simulink library "CRYP_MN_MASTER"  (Simulink 8.6)
settings: Solver=ode45  StartTime=0.0  StopTime=10.0  RelTol=1e-3
libraries: VIS_LIB x19, cdsEpicsOut x16, cdsFilt x12, cdsTP x12, cdsMuxMatrix x6, cdsEpicsBinIn x5, KAGRA_UTIL x1, cdsFunctionCall x1
(part 1 of 2)
settings Model: Creator=controls  LastModifiedBy=controls

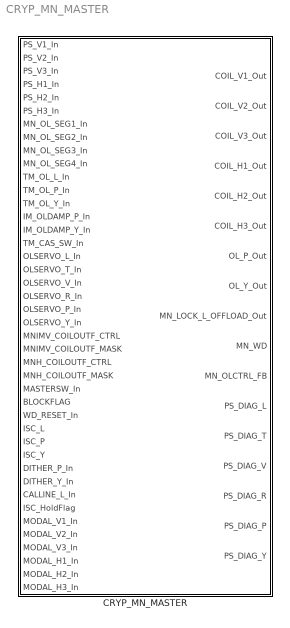
== system CRYP_MN_MASTER ==
  CRYP_MN_MASTER : Subsystem  Description=SIXOSEMSTAGE_FACE_MASTER

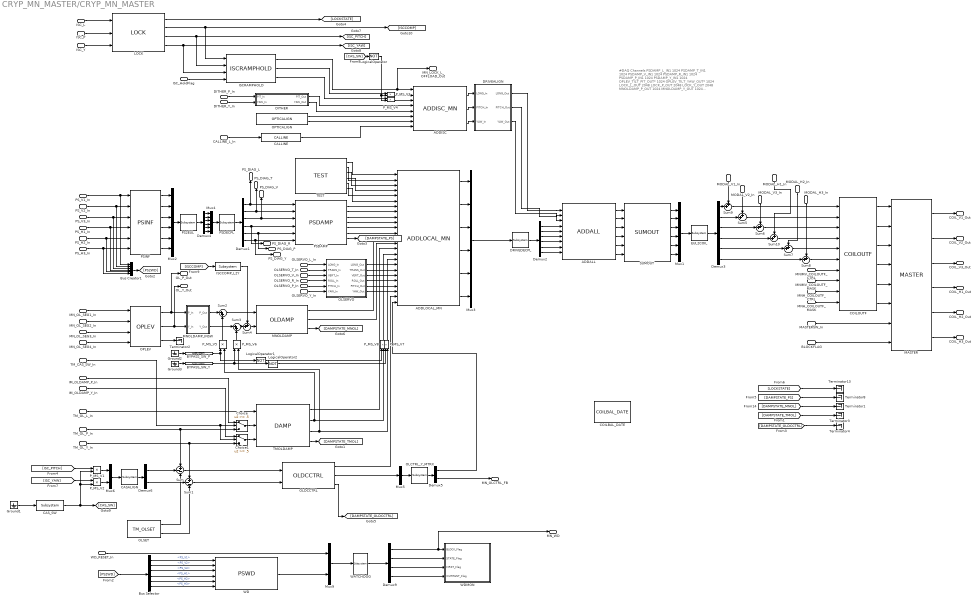
== system CRYP_MN_MASTER/CRYP_MN_MASTER ==
  note: #DAQ Channels
      | PSDAMP_L_IN1 1024
      | PSDAMP_T_IN1 1024
      | PSDAMP_V_IN1 1024
      | PSDAMP_R_IN1 1024
      | PSDAMP_P_IN1 1024
      | PSDAMP_Y_IN1 1024
      | OPLEV_TILT_PIT_OUT* 1024
      | OPLEV_TILT_YAW_OUT* 1024
      | LOCK_L_OUT 2048
      | LOCK_P_OUT 2048
      | LOCK_Y_OUT 2048
      | MNOLDAMP_P_OUT 1024
      | MNOLDAMP_Y_OUT 1024
      | TMOLDAMP_L_OUT 1024
      | TMOLDAMP_P_OUT 1024
      | TMOLDAMP_Y_OUT 1024
      | OLDCCTRL_P_OUT 256
      | OLDCCTRL_Y_OUT 256
      | PSDAMP_L_OUT 1024
      | PSDAMP_T_OUT 1024
      | PSDAMP_V_OUT 1024
      | PSDAMP_R_OUT 1024
      | PSDAMP_P_OUT 1024
      | PSDAMP_Y_OUT 1024
      | SUMOUT_L_OUT 512
      | SUMOUT_T_OUT 512
      | SUMOUT_V_OUT 512
      | SUMOUT_R_OUT 512
      | SUMOUT_P_OUT 512
      | SUMOUT_Y_OUT 512
      | MASTER_OUT_H1 1024
      | MASTER_OUT_H2 1024
      | MASTER_OUT_H3 1024
      | MASTER_OUT_V1 1024
      | MASTER_OUT_V2 1024
      | MASTER_OUT_V3 1024
  PS_V1_In : Inport
  PS_V2_In : Inport  Port=2
  PS_V3_In : Inport  Port=3
  PS_H1_In : Inport  Port=4
  PS_H2_In : Inport  Port=5
  PS_H3_In : Inport  Port=6
  MN_OL_SEG1_In : Inport  Port=7
  MN_OL_SEG2_In : Inport  Port=8
  MN_OL_SEG3_In : Inport  Port=9
  MN_OL_SEG4_In : Inport  Port=10
  TM_OL_L_In : Inport  Port=11
  TM_OL_P_In : Inport  Port=12
  TM_OL_Y_In : Inport  Port=13
  IM_OLDAMP_P_In : Inport  Port=14
  IM_OLDAMP_Y_In : Inport  Port=15
  TM_CAS_SW_In : Inport  Port=16
  OLSERVO_L_In : Inport  Port=17
  OLSERVO_T_In : Inport  Port=18
  OLSERVO_V_In : Inport  Port=19
  OLSERVO_R_In : Inport  Port=20
  OLSERVO_P_In : Inport  Port=21
  OLSERVO_Y_In : Inport  Port=22
  MNIMV_COILOUTF_CTRL : Inport  Port=23
  MNIMV_COILOUTF_MASK : Inport  Port=24
  MNH_COILOUTF_CTRL : Inport  Port=25
  MNH_COILOUTF_MASK : Inport  Port=26
  MASTERSW_In : Inport  Port=27
  BLOCKFLAG : Inport  Port=28
  WD_RESET_In : Inport  Port=29
  ISC_L : Inport  Port=30
  ISC_P : Inport  Port=31
  ISC_Y : Inport  Port=32
  DITHER_P_In : Inport  Port=33
  DITHER_Y_In : Inport  Port=34
  CALLINE_L_In : Inport  Port=35
  ISC_HoldFlag : Inport  Port=36
  MODAL_V1_In : Inport  Port=37
  MODAL_V2_In : Inport  Port=38
  MODAL_V3_In : Inport  Port=39
  MODAL_H1_In : Inport  Port=40
  MODAL_H2_In : Inport  Port=41
  MODAL_H3_In : Inport  Port=42
  ADDALL : VIS_LIB/CrypParts/ADDALL
  ADDISC : VIS_LIB/CrypParts/ADDISC_MN
  ADDLOCAL_MN : VIS_LIB/CrypParts/ADDLOCAL_MN
  BYPASS_SW_P : cdsEpicsBinIn/Subsystem  Tag=cdsEpicsBinIn  Description=|
      | Purpose:                                                                            
      | Create an EPICS binary (0 or 1) input channel to the FE realtime controls.          
      |                                                                                     
      | Operation:                                                                          
      | Outputs value from an EPICS ai record. Value is binary input (bi Epics record type).
      |                                                                                     
      | Usage:                                                                              
      | Name the part with the desired EPICS channel name.
      settings: AttributesFormatString=%<Tag>
  BYPASS_SW_Y : cdsEpicsBinIn/Subsystem  Tag=cdsEpicsBinIn  Description=|
      | Purpose:                                                                            
      | Create an EPICS binary (0 or 1) input channel to the FE realtime controls.          
      |                                                                                     
      | Operation:                                                                          
      | Outputs value from an EPICS ai record. Value is binary input (bi Epics record type).
      |                                                                                     
      | Usage:                                                                              
      | Name the part with the desired EPICS channel name.
      settings: AttributesFormatString=%<Tag>
  Bus Creator1 : BusCreator  Inputs='PS_V1','PS_V2','PS_V3','PS_H1','PS_H2','PS_H3'
  Bus Selector : BusSelector  OutputSignals=PS_V1,PS_V2,PS_V3,PS_H1,PS_H2,PS_H3
  CALLINE : VIS_LIB/CALLINE
  CASALIGN : cdsMuxMatrix/Subsystem  Tag=cdsMuxMatrix  Description=Any size matrix. Inputs and outputs must be connected using Mux and Demux parts.
      settings: AttributesFormatString=%<Tag>
  CAS_SW : cdsEpicsBinIn/Subsystem  Tag=cdsEpicsBinIn  Description=|
      | Purpose:                                                                            
      | Create an EPICS binary (0 or 1) input channel to the FE realtime controls.          
      |                                                                                     
      | Operation:                                                                          
      | Outputs value from an EPICS ai record. Value is binary input (bi Epics record type).
      |                                                                                     
      | Usage:                                                                              
      | Name the part with the desired EPICS channel name.
      settings: AttributesFormatString=%<Tag>
  COILBAL_DATE : VIS_LIB/COILBAL_DATE
  COILOUTF : VIS_LIB/CRYp Blocks/COILOUTF
  Choice : Switch  Threshold=.5
  Choice1 : Switch  Threshold=.5
  DITHER : Subsystem
  DRIVEALIGN : Subsystem
  DRIVEDECPL : cdsMuxMatrix/Subsystem  Tag=cdsMuxMatrix  Description=Any size matrix. Inputs and outputs must be connected using Mux and Demux parts.
      settings: AttributesFormatString=%<Tag>
  Demux{1..4} (4 alike) : Demux  Outputs=6
  Demux5 : Demux  Outputs=2
  Demux6 : Demux  Outputs=2
  Demux9 : Demux
  EUL2COIL : cdsMuxMatrix/Subsystem  Tag=cdsMuxMatrix  Description=Any size matrix. Inputs and outputs must be connected using Mux and Demux parts.
      settings: AttributesFormatString=%<Tag>
  Ground1 : Ground
  Ground2 : Ground
  Ground3 : Ground
  ISCCOMP_L2Y : cdsFilt/Subsystem  Tag=cdsFilt  Description=|
      | Purpose:                                                                                                                                                                                                                                  
      | Standard CDS IIR filter module.                                                                                                                                                                                                           
      |                                                                                                                                                                                                                                           
      | Operation:                                                                                                                                                                                                                                
      | Consists of 10 second order section IIR filters, plus a ramped gain stage. In FE code, also provides pre-defined test points and excitation channel inputs. The filter coefficients are defined in the LIGO system using the 'foton' tool.
      |                                                                                                                                                                                                                                           
      | Usage:                                                                                                                                                                                                                                    
      | Name the part with the desired filter module name.
      settings: AttributesFormatString=%<Tag>
  ISCRAMPHOLD : KAGRA_UTIL/ISCRAMPHOLD
  LOCK : VIS_LIB/CrypParts/LOCK
  LogicalOperator : Logic  Operator=NOT  AllPortsSameDT=off  OutDataTypeStr=boolean
  LogicalOperator1 : Logic  Operator=NOT  AllPortsSameDT=off  OutDataTypeStr=boolean
  LogicalOperator2 : Logic  Operator=NOT  AllPortsSameDT=off  OutDataTypeStr=boolean
  MASTER : VIS_LIB/CRYp Blocks/MASTER
  MNOLDAMP : VIS_LIB/OLDAMP
  MNOLDAMP_INSW : Subsystem
  Mux{1..4} (4 alike) : Mux  Inputs=6
  Mux5 : Mux  Inputs=1
  Mux6 : Mux  Inputs=2
  Mux9 : Mux  Inputs=2
  OLCTRL_Y_MTRX : cdsMuxMatrix/Subsystem  Tag=cdsMuxMatrix  Description=Any size matrix. Inputs and outputs must be connected using Mux and Demux parts.
      settings: AttributesFormatString=%<Tag>
  OLDCCTRL : VIS_LIB/CrypParts/OLDCCTRL
  OLSERVO : Subsystem
  OLSET : VIS_LIB/CrypParts/TM_OLSET
  OPLEV : VIS_LIB/CrypParts/OPLEV
  OPTICALIGN : VIS_LIB/CrypParts/OPTICALIGN
  PS2EUL : cdsMuxMatrix/Subsystem  Tag=cdsMuxMatrix  Description=Any size matrix. Inputs and outputs must be connected using Mux and Demux parts.
      settings: AttributesFormatString=%<Tag>
  PSDAMP : VIS_LIB/CrypParts/PSDAMP
  PSDECPL : cdsMuxMatrix/Subsystem  Tag=cdsMuxMatrix  Description=Any size matrix. Inputs and outputs must be connected using Mux and Demux parts.
      settings: AttributesFormatString=%<Tag>
  PSINF : VIS_LIB/CrypParts/PSINF
  P_MS_V{1..8} (8 alike) : Product  RndMeth=Zero
  SUMOUT : VIS_LIB/CrypParts/SUMOUT
  Sum : Sum  Inputs=+--
  Sum1 : Sum  Inputs=+--
  Sum{4..10} (7 alike) : Sum  Inputs=++|
  Sum2 : Sum  Inputs=|++
  Sum3 : Sum  Inputs=|++
  TEST : VIS_LIB/CrypParts/TEST
  TMOLDAMP : VIS_LIB/CrypParts/DAMP
  Terminator{1..4,8,13} (6 alike) : Terminator
  WATCHDOG : cdsFunctionCall/Subsystem  Tag=cdsFunctionCall  Description=inline OSEMWATCHDOG /opt/rtcds/userapps/release/vis/common/src/WATCHDOG.c
      settings: AttributesFormatString=%<Tag>\n%<Description>
  WD : VIS_LIB/CRYp Blocks/PSWD
  WDMON : Subsystem
  COIL_V1_Out : Outport
  COIL_V2_Out : Outport  Port=2
  COIL_V3_Out : Outport  Port=3
  COIL_H1_Out : Outport  Port=4
  COIL_H2_Out : Outport  Port=5
  COIL_H3_Out : Outport  Port=6
  OL_P_Out : Outport  Port=7
  OL_Y_Out : Outport  Port=8
  MN_LOCK_L_OFFLOAD_Out : Outport  Port=9
  MN_WD : Outport  Port=10
  MN_OLCTRL_FB : Outport  Port=11
  PS_DIAG_L : Outport  Port=12
  PS_DIAG_T : Outport  Port=13
  PS_DIAG_V : Outport  Port=14
  PS_DIAG_R : Outport  Port=15
  PS_DIAG_P : Outport  Port=16
  PS_DIAG_Y : Outport  Port=17
  wires:
  Demux3/6 -> Sum8/2
  MODAL_H3_In/1 -> Sum8/1
  Sum8/1 -> COILOUTF/6
  Demux3/5 -> Sum7/2
  MODAL_H2_In/1 -> Sum7/1
  Sum7/1 -> COILOUTF/5
  Demux3/4 -> Sum10/2
  MODAL_H1_In/1 -> Sum10/1
  Sum10/1 -> COILOUTF/4
  Demux3/3 -> Sum6/2
  MODAL_V3_In/1 -> Sum6/1
  Sum6/1 -> COILOUTF/3
  Demux3/2 -> Sum5/2
  MODAL_V2_In/1 -> Sum5/1
  Sum5/1 -> COILOUTF/2
  Demux3/1 -> Sum9/2
  MODAL_V1_In/1 -> Sum9/1
  Sum9/1 -> COILOUTF/1
  Demux1/1 -> PSDAMP/1, PS_DIAG_L/1
  Demux1/2 -> PSDAMP/2, PS_DIAG_T/1
  Demux1/5 -> PSDAMP/5, PS_DIAG_P/1
  Demux1/6 -> PSDAMP/6, PS_DIAG_Y/1
  ADDLOCAL_MN/6 -> Mux3/6
  ADDLOCAL_MN/5 -> Mux3/5
  ADDLOCAL_MN/4 -> Mux3/4
  ADDLOCAL_MN/3 -> Mux3/3
  ADDLOCAL_MN/2 -> Mux3/2
  ADDLOCAL_MN/1 -> Mux3/1
  ISC_HoldFlag/1 -> ISCRAMPHOLD/4
  ISCRAMPHOLD/3 -> P_MS_V4/1
  ISCRAMPHOLD/2 -> P_MS_V3/1
  ISCRAMPHOLD/1 -> ADDISC/1, MN_LOCK_L_OFFLOAD_Out/1
  MNOLDAMP_INSW/2(Y_Out) -> Sum3/1
  MNOLDAMP_INSW/1(P_Out) -> Sum2/1
  P_MS_V7/1 -> ADDLOCAL_MN/17
  P_MS_V8/1 -> ADDLOCAL_MN/16
  LogicalOperator1/1 -> P_MS_V8/1
  TM_CAS_SW_In/1 -> Choice/2, Choice1/2
  IM_OLDAMP_Y_In/1 -> Choice1/1
  IM_OLDAMP_P_In/1 -> Choice/1
  P_MS_V6/1 -> Sum3/2
  P_MS_V5/1 -> Sum2/2
  Sum2/1 -> MNOLDAMP/1
  Choice1/1 -> TMOLDAMP/3
  Choice/1 -> TMOLDAMP/2
  OLSET/2 -> Sum1/3
  OLSET/1 -> Sum/3
  Demux6/2 -> Sum1/2
  Demux6/1 -> Sum/2
  LogicalOperator/1 -> P_MS_V4/2, P_MS_V3/2
  P_MS_V3/1 -> ADDISC/2
  P_MS_V4/1 -> ADDISC/3
  DRIVEALIGN/3(YAW_Out) -> ADDALL/3
  DRIVEALIGN/2(PITCH_Out) -> ADDALL/2
  [CAS_SW] -> LogicalOperator/1
  CASALIGN/1 -> Demux6/1
  Mux6/1 -> CASALIGN/1
  P_MS_V2/1 -> Mux6/2
  P_MS_V1/1 -> Mux6/1
  CAS_SW/1 -> P_MS_V2/2, P_MS_V1/2, [CAS_SW]
  [ISC_PITCH] -> P_MS_V1/1
  [ISC_YAW] -> P_MS_V2/1
  Ground1/1 -> CAS_SW/1
  Demux5/1 -> ADDLOCAL_MN/25
  OLDCCTRL/2 -> Mux5/1
  Demux5/2 -> MN_OLCTRL_FB/1
  OLCTRL_Y_MTRX/1 -> Demux5/1
  Mux5/1 -> OLCTRL_Y_MTRX/1
  Sum1/1 -> OLDCCTRL/2
  Sum/1 -> OLDCCTRL/1
  [DAMPSTATE_OLDCCTRL] -> Terminator4/1
  OLDCCTRL/1 -> ADDLOCAL_MN/24
  TEST/6 -> ADDLOCAL_MN/6
  TEST/5 -> ADDLOCAL_MN/5
  TEST/4 -> ADDLOCAL_MN/4
  TEST/3 -> ADDLOCAL_MN/3
  TEST/2 -> ADDLOCAL_MN/2
  TEST/1 -> ADDLOCAL_MN/1
  OLDCCTRL/3 -> [DAMPSTATE_OLDCCTRL]
  OLSERVO/3(VERT_Out) -> ADDLOCAL_MN/20
  OLSERVO/2(TRANS_Out) -> ADDLOCAL_MN/19
  OLSERVO/1(LONG_Out) -> ADDLOCAL_MN/18
  OLSERVO/6(YAW_Out) -> ADDLOCAL_MN/23
  OLSERVO/5(PITCH_Out) -> ADDLOCAL_MN/22
  OLSERVO/4(ROLL_Out) -> ADDLOCAL_MN/21
  OLSERVO_Y_In/1 -> OLSERVO/6(YAW_In)
  OLSERVO_P_In/1 -> OLSERVO/5(PITCH_In)
  OLSERVO_R_In/1 -> OLSERVO/4(ROLL_In)
  OLSERVO_V_In/1 -> OLSERVO/3(VERT_In)
  OLSERVO_T_In/1 -> OLSERVO/2(TRANS_In)
  OLSERVO_L_In/1 -> OLSERVO/1(LONG_In)
  PSDECPL/1 -> Demux1/1
  Mux4/1 -> PSDECPL/1
  Demux4/6 -> Mux4/6
  Demux4/5 -> Mux4/5
  Demux4/4 -> Mux4/4
  Demux4/3 -> Mux4/3
  Demux4/2 -> Mux4/2
  Demux4/1 -> Mux4/1
  PS2EUL/1 -> Demux4/1
  SUMOUT/6 -> Mux1/6
  SUMOUT/5 -> Mux1/5
  SUMOUT/4 -> Mux1/4
  SUMOUT/3 -> Mux1/3
  SUMOUT/2 -> Mux1/2
  SUMOUT/1 -> Mux1/1
  ADDALL/6 -> SUMOUT/6
  ADDALL/5 -> SUMOUT/5
  ADDALL/4 -> SUMOUT/4
  ADDALL/3 -> SUMOUT/3
  ADDALL/2 -> SUMOUT/2
  ADDALL/1 -> SUMOUT/1
  TM_OL_Y_In/1 -> Choice1/3, Sum1/1
  TM_OL_P_In/1 -> Sum/1, Choice/3
  TM_OL_L_In/1 -> TMOLDAMP/1
  [DAMPSTATE_TMOL] -> Terminator3/1
  TMOLDAMP/4 -> [DAMPSTATE_TMOL]
  Demux2/3 -> ADDALL/6
  Demux2/5 -> ADDALL/8
  Demux2/4 -> ADDALL/7
  Demux2/2 -> ADDALL/5
  Demux2/6 -> ADDALL/9
  Demux2/1 -> ADDALL/4
  DRIVEDECPL/1 -> Demux2/1
  Mux3/1 -> DRIVEDECPL/1
  DRIVEALIGN/1(LONG_Out) -> ADDALL/1
  TMOLDAMP/1 -> ADDLOCAL_MN/15
  TMOLDAMP/2 -> P_MS_V5/2, P_MS_V8/2
  TMOLDAMP/3 -> P_MS_V6/2, P_MS_V7/2
  MNOLDAMP/1 -> ADDLOCAL_MN/13
  MNOLDAMP/2 -> ADDLOCAL_MN/14
  PSDAMP/6 -> ADDLOCAL_MN/12
  PSDAMP/5 -> ADDLOCAL_MN/11
  PSDAMP/4 -> ADDLOCAL_MN/10
  PSDAMP/3 -> ADDLOCAL_MN/9
  PSDAMP/2 -> ADDLOCAL_MN/8
  PSDAMP/1 -> ADDLOCAL_MN/7
  ADDISC/1 -> DRIVEALIGN/1(LONG_In)
  ADDISC/2 -> DRIVEALIGN/2(PITCH_In)
  ADDISC/3 -> DRIVEALIGN/3(YAW_In)
  OPTICALIGN/2 -> ADDISC/7
  OPTICALIGN/1 -> ADDISC/6
  DITHER/2(YAW_Out) -> ADDISC/5
  DITHER/1(PIT_Out) -> ADDISC/4
  LOCK/2 -> [ISCCOMP], ISCRAMPHOLD/1
  LOCK/3 -> [ISC_PITCH], ISCRAMPHOLD/2
  LOCK/4 -> [ISC_YAW], ISCRAMPHOLD/3
  BLOCKFLAG/1 -> MASTER/8
  Mux1/1 -> EUL2COIL/1
  Bus Selector/1 -> WD/1  "<PS_V1>"
  Bus Selector/3 -> WD/3  "<PS_V3>"
  Bus Selector/4 -> WD/4  "<PS_H1>"
  Bus Selector/5 -> WD/5  "<PS_H2>"
  Bus Selector/2 -> WD/2  "<PS_V2>"
  Bus Selector/6 -> WD/6  "<PS_H3>"
  OPLEV/3 -> Terminator2/1
  OPLEV/2 -> OL_Y_Out/1, MNOLDAMP_INSW/2(Y_In)
  OPLEV/1 -> MNOLDAMP_INSW/1(P_In), OL_P_Out/1
  MN_OL_SEG1_In/1 -> OPLEV/1
  MN_OL_SEG2_In/1 -> OPLEV/2
  MN_OL_SEG3_In/1 -> OPLEV/3
  MN_OL_SEG4_In/1 -> OPLEV/4
  ISC_L/1 -> LOCK/1
  ISC_Y/1 -> LOCK/3
  ISC_P/1 -> LOCK/2
  Demux1/3 -> PSDAMP/3, PS_DIAG_V/1
  Demux1/4 -> PSDAMP/4, PS_DIAG_R/1
  PSINF/5 -> Mux2/5
  PSINF/4 -> Mux2/4
  PSINF/3 -> Mux2/3
  PSINF/2 -> Mux2/2
  PSINF/1 -> Mux2/1
  PSINF/6 -> Mux2/6
  MASTER/3 -> COIL_V3_Out/1
  MASTER/6 -> COIL_H3_Out/1
  MASTER/5 -> COIL_H2_Out/1
  MASTER/4 -> COIL_H1_Out/1
  MASTER/2 -> COIL_V2_Out/1
  MASTER/1 -> COIL_V1_Out/1
  MASTERSW_In/1 -> MASTER/7
  COILOUTF/6 -> MASTER/6
  COILOUTF/5 -> MASTER/5
  COILOUTF/4 -> MASTER/4
  COILOUTF/3 -> MASTER/3
  COILOUTF/1 -> MASTER/1
  COILOUTF/2 -> MASTER/2
  MNH_COILOUTF_CTRL/1 -> COILOUTF/9
  MNIMV_COILOUTF_MASK/1 -> COILOUTF/8
  MNH_COILOUTF_MASK/1 -> COILOUTF/10
  MNIMV_COILOUTF_CTRL/1 -> COILOUTF/7
  PS_V3_In/1 -> PSINF/3, Bus Creator1/3
  PS_H1_In/1 -> PSINF/4, Bus Creator1/4
  PS_V2_In/1 -> PSINF/2, Bus Creator1/2
  PS_V1_In/1 -> Bus Creator1/1, PSINF/1
  PS_H3_In/1 -> PSINF/6, Bus Creator1/6
  PS_H2_In/1 -> PSINF/5, Bus Creator1/5
  [DAMPSTATE_MNOL] -> Terminator1/1
  MNOLDAMP/3 -> [DAMPSTATE_MNOL]
  DITHER_P_In/1 -> DITHER/1(PIT_In)
  DITHER_Y_In/1 -> DITHER/2(YAW_In)
  WD_RESET_In/1 -> Mux9/1
  WD/1 -> Mux9/2
  [LOCKSTATE] -> Terminator13/1
  LOCK/1 -> [LOCKSTATE]
  [DAMPSTATE_PS] -> Terminator8/1
  PSDAMP/7 -> [DAMPSTATE_PS]
  Demux9/1 -> WDMON/1(BLOCK_Flag), MN_WD/1
  Mux2/1 -> PS2EUL/1
  Bus Creator1/1 -> [PS2WD]
  [PS2WD] -> Bus Selector/1
  EUL2COIL/1 -> Demux3/1
  Demux9/2 -> WDMON/2(STATE_Flag)
  Demux9/3 -> WDMON/3(FIRST_Flag)
  Demux9/4 -> WDMON/4(CURRENT_Flag)
  Mux9/1 -> WATCHDOG/1
  WATCHDOG/1 -> Demux9/1
  Ground2/1 -> BYPASS_SW_P/1
  BYPASS_SW_P/1 -> LogicalOperator1/1, P_MS_V5/1
  LogicalOperator2/1 -> P_MS_V7/1
  BYPASS_SW_Y/1 -> P_MS_V6/1, LogicalOperator2/1
  Ground3/1 -> BYPASS_SW_Y/1
  Sum3/1 -> Sum4/2
  Sum4/1 -> MNOLDAMP/2
  ISCCOMP_L2Y/1 -> Sum4/1
  [ISCCOMP] -> ISCCOMP_L2Y/1
  CALLINE/1 -> ADDISC/8
  CALLINE_L_In/1 -> CALLINE/1

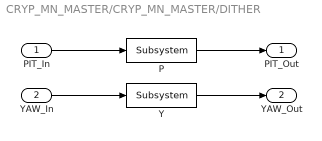
== system CRYP_MN_MASTER/CRYP_MN_MASTER/DITHER ==
  PIT_In : Inport
  YAW_In : Inport  Port=2
  P : cdsFilt/Subsystem  Tag=cdsFilt  Description=|
      | Purpose:                                                                                                                                                                                                                                  
      | Standard CDS IIR filter module.                                                                                                                                                                                                           
      |                                                                                                                                                                                                                                           
      | Operation:                                                                                                                                                                                                                                
      | Consists of 10 second order section IIR filters, plus a ramped gain stage. In FE code, also provides pre-defined test points and excitation channel inputs. The filter coefficients are defined in the LIGO system using the 'foton' tool.
      |                                                                                                                                                                                                                                           
      | Usage:                                                                                                                                                                                                                                    
      | Name the part with the desired filter module name.
      settings: AttributesFormatString=%<Tag>
  Y : cdsFilt/Subsystem  Tag=cdsFilt  Description=|
      | Purpose:                                                                                                                                                                                                                                  
      | Standard CDS IIR filter module.                                                                                                                                                                                                           
      |                                                                                                                                                                                                                                           
      | Operation:                                                                                                                                                                                                                                
      | Consists of 10 second order section IIR filters, plus a ramped gain stage. In FE code, also provides pre-defined test points and excitation channel inputs. The filter coefficients are defined in the LIGO system using the 'foton' tool.
      |                                                                                                                                                                                                                                           
      | Usage:                                                                                                                                                                                                                                    
      | Name the part with the desired filter module name.
      settings: AttributesFormatString=%<Tag>
  PIT_Out : Outport
  YAW_Out : Outport  Port=2
  wires:
  P/1 -> PIT_Out/1
  YAW_In/1 -> Y/1
  Y/1 -> YAW_Out/1
  PIT_In/1 -> P/1

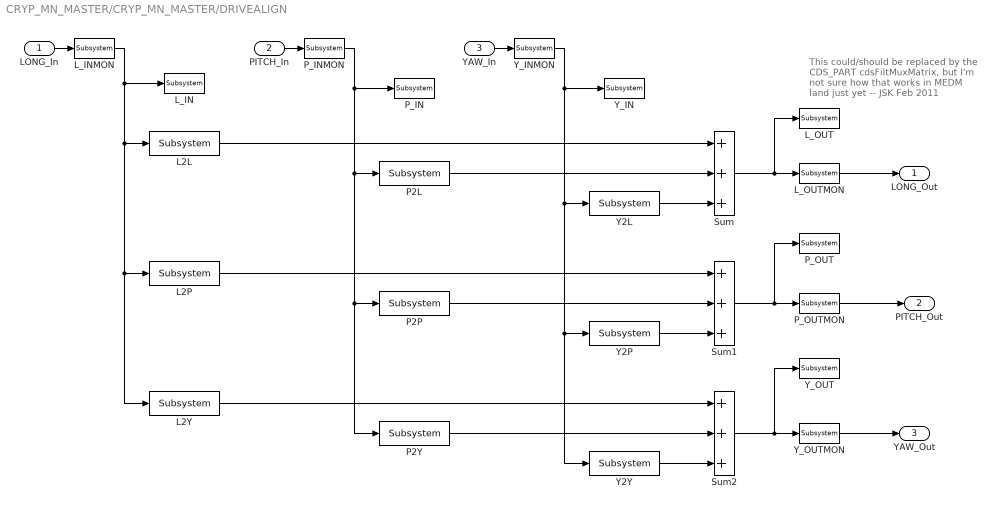
== system CRYP_MN_MASTER/CRYP_MN_MASTER/DRIVEALIGN ==
  note: This could/should be replaced by
      | the CDS_PART cdsFiltMuxMatrix,
      | but I'm not sure how that works
      | in MEDM land just yet
      | -- JSK Feb 2011
  LONG_In : Inport
  PITCH_In : Inport  Port=2
  YAW_In : Inport  Port=3
  L2L : cdsFilt/Subsystem  Tag=cdsFilt  Description=|
      | Purpose:                                                                                                                                                                                                                                  
      | Standard CDS IIR filter module.                                                                                                                                                                                                           
      |                                                                                                                                                                                                                                           
      | Operation:                                                                                                                                                                                                                                
      | Consists of 10 second order section IIR filters, plus a ramped gain stage. In FE code, also provides pre-defined test points and excitation channel inputs. The filter coefficients are defined in the LIGO system using the 'foton' tool.
      |                                                                                                                                                                                                                                           
      | Usage:                                                                                                                                                                                                                                    
      | Name the part with the desired filter module name.
      settings: AttributesFormatString=%<Tag>
  L2P : cdsFilt/Subsystem  Tag=cdsFilt  Description=|
      | Purpose:                                                                                                                                                                                                                                  
      | Standard CDS IIR filter module.                                                                                                                                                                                                           
      |                                                                                                                                                                                                                                           
      | Operation:                                                                                                                                                                                                                                
      | Consists of 10 second order section IIR filters, plus a ramped gain stage. In FE code, also provides pre-defined test points and excitation channel inputs. The filter coefficients are defined in the LIGO system using the 'foton' tool.
      |                                                                                                                                                                                                                                           
      | Usage:                                                                                                                                                                                                                                    
      | Name the part with the desired filter module name.
      settings: AttributesFormatString=%<Tag>
  L2Y : cdsFilt/Subsystem  Tag=cdsFilt  Description=|
      | Purpose:                                                                                                                                                                                                                                  
      | Standard CDS IIR filter module.                                                                                                                                                                                                           
      |                                                                                                                                                                                                                                           
      | Operation:                                                                                                                                                                                                                                
      | Consists of 10 second order section IIR filters, plus a ramped gain stage. In FE code, also provides pre-defined test points and excitation channel inputs. The filter coefficients are defined in the LIGO system using the 'foton' tool.
      |                                                                                                                                                                                                                                           
      | Usage:                                                                                                                                                                                                                                    
      | Name the part with the desired filter module name.
      settings: AttributesFormatString=%<Tag>
  L_IN : cdsTP/Subsystem  Tag=Test Point
      settings: AttributesFormatString=%<Tag>
  L_INMON : cdsEpicsOut/Subsystem  Tag=cdsEpicsOutput  Description=|
      | Purpose:                                          
      | Output a FE signal to an EPICS channel.           
      |                                                   
      | Operation:                                        
      | Takes input value and passes it to EPICS record.  
      |                                                   
      | Usage:                                            
      | Name the part with the desired EPICS rrecord name.
      settings: AttributesFormatString=%<Tag>
  L_OUT : cdsTP/Subsystem  Tag=Test Point
      settings: AttributesFormatString=%<Tag>
  L_OUTMON : cdsEpicsOut/Subsystem  Tag=cdsEpicsOutput  Description=|
      | Purpose:                                          
      | Output a FE signal to an EPICS channel.           
      |                                                   
      | Operation:                                        
      | Takes input value and passes it to EPICS record.  
      |                                                   
      | Usage:                                            
      | Name the part with the desired EPICS rrecord name.
      settings: AttributesFormatString=%<Tag>
  P2L : cdsFilt/Subsystem  Tag=cdsFilt  Description=|
      | Purpose:                                                                                                                                                                                                                                  
      | Standard CDS IIR filter module.                                                                                                                                                                                                           
      |                                                                                                                                                                                                                                           
      | Operation:                                                                                                                                                                                                                                
      | Consists of 10 second order section IIR filters, plus a ramped gain stage. In FE code, also provides pre-defined test points and excitation channel inputs. The filter coefficients are defined in the LIGO system using the 'foton' tool.
      |                                                                                                                                                                                                                                           
      | Usage:                                                                                                                                                                                                                                    
      | Name the part with the desired filter module name.
      settings: AttributesFormatString=%<Tag>
  P2P : cdsFilt/Subsystem  Tag=cdsFilt  Description=|
      | Purpose:                                                                                                                                                                                                                                  
      | Standard CDS IIR filter module.                                                                                                                                                                                                           
      |                                                                                                                                                                                                                                           
      | Operation:                                                                                                                                                                                                                                
      | Consists of 10 second order section IIR filters, plus a ramped gain stage. In FE code, also provides pre-defined test points and excitation channel inputs. The filter coefficients are defined in the LIGO system using the 'foton' tool.
      |                                                                                                                                                                                                                                           
      | Usage:                                                                                                                                                                                                                                    
      | Name the part with the desired filter module name.
      settings: AttributesFormatString=%<Tag>
  P2Y : cdsFilt/Subsystem  Tag=cdsFilt  Description=|
      | Purpose:                                                                                                                                                                                                                                  
      | Standard CDS IIR filter module.                                                                                                                                                                                                           
      |                                                                                                                                                                                                                                           
      | Operation:                                                                                                                                                                                                                                
      | Consists of 10 second order section IIR filters, plus a ramped gain stage. In FE code, also provides pre-defined test points and excitation channel inputs. The filter coefficients are defined in the LIGO system using the 'foton' tool.
      |                                                                                                                                                                                                                                           
      | Usage:                                                                                                                                                                                                                                    
      | Name the part with the desired filter module name.
      settings: AttributesFormatString=%<Tag>
  P_IN : cdsTP/Subsystem  Tag=Test Point
      settings: AttributesFormatString=%<Tag>
  P_INMON : cdsEpicsOut/Subsystem  Tag=cdsEpicsOutput  Description=|
      | Purpose:                                          
      | Output a FE signal to an EPICS channel.           
      |                                                   
      | Operation:                                        
      | Takes input value and passes it to EPICS record.  
      |                                                   
      | Usage:                                            
      | Name the part with the desired EPICS rrecord name.
      settings: AttributesFormatString=%<Tag>
  P_OUT : cdsTP/Subsystem  Tag=Test Point
      settings: AttributesFormatString=%<Tag>
  P_OUTMON : cdsEpicsOut/Subsystem  Tag=cdsEpicsOutput  Description=|
      | Purpose:                                          
      | Output a FE signal to an EPICS channel.           
      |                                                   
      | Operation:                                        
      | Takes input value and passes it to EPICS record.  
      |                                                   
      | Usage:                                            
      | Name the part with the desired EPICS rrecord name.
      settings: AttributesFormatString=%<Tag>
  Sum : Sum  Inputs=+++
  Sum1 : Sum  Inputs=+++
  Sum2 : Sum  Inputs=+++
  Y2L : cdsFilt/Subsystem  Tag=cdsFilt  Description=|
      | Purpose:                                                                                                                                                                                                                                  
      | Standard CDS IIR filter module.                                                                                                                                                                                                           
      |                                                                                                                                                                                                                                           
      | Operation:                                                                                                                                                                                                                                
      | Consists of 10 second order section IIR filters, plus a ramped gain stage. In FE code, also provides pre-defined test points and excitation channel inputs. The filter coefficients are defined in the LIGO system using the 'foton' tool.
      |                                                                                                                                                                                                                                           
      | Usage:                                                                                                                                                                                                                                    
      | Name the part with the desired filter module name.
      settings: AttributesFormatString=%<Tag>
  Y2P : cdsFilt/Subsystem  Tag=cdsFilt  Description=|
      | Purpose:                                                                                                                                                                                                                                  
      | Standard CDS IIR filter module.                                                                                                                                                                                                           
      |                                                                                                                                                                                                                                           
      | Operation:                                                                                                                                                                                                                                
      | Consists of 10 second order section IIR filters, plus a ramped gain stage. In FE code, also provides pre-defined test points and excitation channel inputs. The filter coefficients are defined in the LIGO system using the 'foton' tool.
      |                                                                                                                                                                                                                                           
      | Usage:                                                                                                                                                                                                                                    
      | Name the part with the desired filter module name.
      settings: AttributesFormatString=%<Tag>
  Y2Y : cdsFilt/Subsystem  Tag=cdsFilt  Description=|
      | Purpose:                                                                                                                                                                                                                                  
      | Standard CDS IIR filter module.                                                                                                                                                                                                           
      |                                                                                                                                                                                                                                           
      | Operation:                                                                                                                                                                                                                                
      | Consists of 10 second order section IIR filters, plus a ramped gain stage. In FE code, also provides pre-defined test points and excitation channel inputs. The filter coefficients are defined in the LIGO system using the 'foton' tool.
      |                                                                                                                                                                                                                                           
      | Usage:                                                                                                                                                                                                                                    
      | Name the part with the desired filter module name.
      settings: AttributesFormatString=%<Tag>
  Y_IN : cdsTP/Subsystem  Tag=Test Point
      settings: AttributesFormatString=%<Tag>
  Y_INMON : cdsEpicsOut/Subsystem  Tag=cdsEpicsOutput  Description=|
      | Purpose:                                          
      | Output a FE signal to an EPICS channel.           
      |                                                   
      | Operation:                                        
      | Takes input value and passes it to EPICS record.  
      |                                                   
      | Usage:                                            
      | Name the part with the desired EPICS rrecord name.
      settings: AttributesFormatString=%<Tag>
  Y_OUT : cdsTP/Subsystem  Tag=Test Point
      settings: AttributesFormatString=%<Tag>
  Y_OUTMON : cdsEpicsOut/Subsystem  Tag=cdsEpicsOutput  Description=|
      | Purpose:                                          
      | Output a FE signal to an EPICS channel.           
      |                                                   
      | Operation:                                        
      | Takes input value and passes it to EPICS record.  
      |                                                   
      | Usage:                                            
      | Name the part with the desired EPICS rrecord name.
      settings: AttributesFormatString=%<Tag>
  LONG_Out : Outport
  PITCH_Out : Outport  Port=2
  YAW_Out : Outport  Port=3
  wires:
  Y_OUTMON/1 -> YAW_Out/1
  P_OUTMON/1 -> PITCH_Out/1
  L_OUTMON/1 -> LONG_Out/1
  Y_INMON/1 -> Y_IN/1, Y2L/1, Y2Y/1, Y2P/1
  P_INMON/1 -> P_IN/1, P2L/1, P2Y/1, P2P/1
  L_INMON/1 -> L_IN/1, L2Y/1, L2P/1, L2L/1
  L2L/1 -> Sum/1
  P2L/1 -> Sum/2
  Y2L/1 -> Sum/3
  Y2P/1 -> Sum1/3
  P2P/1 -> Sum1/2
  L2P/1 -> Sum1/1
  Y2Y/1 -> Sum2/3
  P2Y/1 -> Sum2/2
  L2Y/1 -> Sum2/1
  Sum/1 -> L_OUT/1, L_OUTMON/1
  Sum1/1 -> P_OUT/1, P_OUTMON/1
  Sum2/1 -> Y_OUT/1, Y_OUTMON/1
  LONG_In/1 -> L_INMON/1
  PITCH_In/1 -> P_INMON/1
  YAW_In/1 -> Y_INMON/1

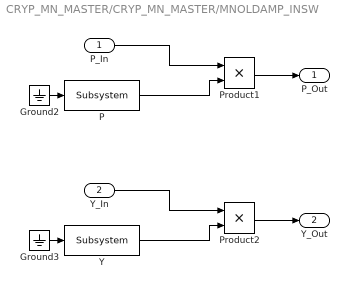
== system CRYP_MN_MASTER/CRYP_MN_MASTER/MNOLDAMP_INSW ==
  P_In : Inport
  Y_In : Inport  Port=2
  Ground2 : Ground
  Ground3 : Ground
  P : cdsEpicsBinIn/Subsystem  Tag=cdsEpicsBinIn  Description=|
      | Purpose:                                                                            
      | Create an EPICS binary (0 or 1) input channel to the FE realtime controls.          
      |                                                                                     
      | Operation:                                                                          
      | Outputs value from an EPICS ai record. Value is binary input (bi Epics record type).
      |                                                                                     
      | Usage:                                                                              
      | Name the part with the desired EPICS channel name.
      settings: AttributesFormatString=%<Tag>
  Product1 : Product  RndMeth=Zero
  Product2 : Product  RndMeth=Zero
  Y : cdsEpicsBinIn/Subsystem  Tag=cdsEpicsBinIn  Description=|
      | Purpose:                                                                            
      | Create an EPICS binary (0 or 1) input channel to the FE realtime controls.          
      |                                                                                     
      | Operation:                                                                          
      | Outputs value from an EPICS ai record. Value is binary input (bi Epics record type).
      |                                                                                     
      | Usage:                                                                              
      | Name the part with the desired EPICS channel name.
      settings: AttributesFormatString=%<Tag>
  P_Out : Outport
  Y_Out : Outport  Port=2
  wires:
  Ground2/1 -> P/1
  P/1 -> Product1/2
  P_In/1 -> Product1/1
  Product1/1 -> P_Out/1
  Ground3/1 -> Y/1
  Y/1 -> Product2/2
  Y_In/1 -> Product2/1
  Product2/1 -> Y_Out/1

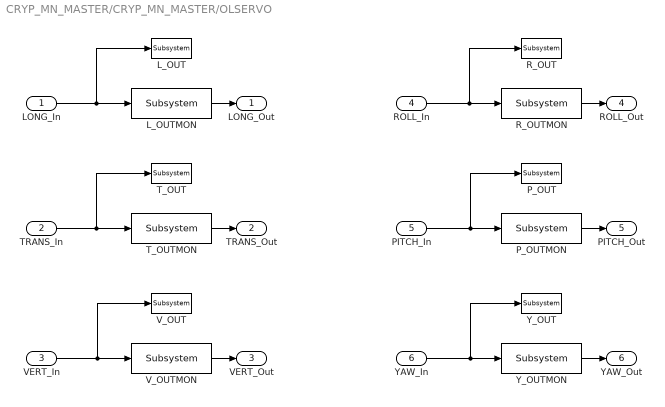
== system CRYP_MN_MASTER/CRYP_MN_MASTER/OLSERVO ==
  LONG_In : Inport
  TRANS_In : Inport  Port=2
  VERT_In : Inport  Port=3
  ROLL_In : Inport  Port=4
  PITCH_In : Inport  Port=5
  YAW_In : Inport  Port=6
  L_OUT : cdsTP/Subsystem  Tag=Test Point
      settings: AttributesFormatString=%<Tag>
  L_OUTMON : cdsEpicsOut/Subsystem  Tag=cdsEpicsOutput  Description=|
      | Purpose:                                          
      | Output a FE signal to an EPICS channel.           
      |                                                   
      | Operation:                                        
      | Takes input value and passes it to EPICS record.  
      |                                                   
      | Usage:                                            
      | Name the part with the desired EPICS rrecord name.
      settings: AttributesFormatString=%<Tag>
  P_OUT : cdsTP/Subsystem  Tag=Test Point
      settings: AttributesFormatString=%<Tag>
  P_OUTMON : cdsEpicsOut/Subsystem  Tag=cdsEpicsOutput  Description=|
      | Purpose:                                          
      | Output a FE signal to an EPICS channel.           
      |                                                   
      | Operation:                                        
      | Takes input value and passes it to EPICS record.  
      |                                                   
      | Usage:                                            
      | Name the part with the desired EPICS rrecord name.
      settings: AttributesFormatString=%<Tag>
  R_OUT : cdsTP/Subsystem  Tag=Test Point
      settings: AttributesFormatString=%<Tag>
  R_OUTMON : cdsEpicsOut/Subsystem  Tag=cdsEpicsOutput  Description=|
      | Purpose:                                          
      | Output a FE signal to an EPICS channel.           
      |                                                   
      | Operation:                                        
      | Takes input value and passes it to EPICS record.  
      |                                                   
      | Usage:                                            
      | Name the part with the desired EPICS rrecord name.
      settings: AttributesFormatString=%<Tag>
  T_OUT : cdsTP/Subsystem  Tag=Test Point
      settings: AttributesFormatString=%<Tag>
  T_OUTMON : cdsEpicsOut/Subsystem  Tag=cdsEpicsOutput  Description=|
      | Purpose:                                          
      | Output a FE signal to an EPICS channel.           
      |                                                   
      | Operation:                                        
      | Takes input value and passes it to EPICS record.  
      |                                                   
      | Usage:                                            
      | Name the part with the desired EPICS rrecord name.
      settings: AttributesFormatString=%<Tag>
  V_OUT : cdsTP/Subsystem  Tag=Test Point
      settings: AttributesFormatString=%<Tag>
  V_OUTMON : cdsEpicsOut/Subsystem  Tag=cdsEpicsOutput  Description=|
      | Purpose:                                          
      | Output a FE signal to an EPICS channel.           
      |                                                   
      | Operation:                                        
      | Takes input value and passes it to EPICS record.  
      |                                                   
      | Usage:                                            
      | Name the part with the desired EPICS rrecord name.
      settings: AttributesFormatString=%<Tag>
  Y_OUT : cdsTP/Subsystem  Tag=Test Point
      settings: AttributesFormatString=%<Tag>
  Y_OUTMON : cdsEpicsOut/Subsystem  Tag=cdsEpicsOutput  Description=|
      | Purpose:                                          
      | Output a FE signal to an EPICS channel.           
      |                                                   
      | Operation:                                        
      | Takes input value and passes it to EPICS record.  
      |                                                   
      | Usage:                                            
      | Name the part with the desired EPICS rrecord name.
      settings: AttributesFormatString=%<Tag>
  LONG_Out : Outport
  TRANS_Out : Outport  Port=2
  VERT_Out : Outport  Port=3
  ROLL_Out : Outport  Port=4
  PITCH_Out : Outport  Port=5
  YAW_Out : Outport  Port=6
  wires:
  YAW_In/1 -> Y_OUTMON/1, Y_OUT/1
  Y_OUTMON/1 -> YAW_Out/1
  PITCH_In/1 -> P_OUTMON/1, P_OUT/1
  P_OUTMON/1 -> PITCH_Out/1
  VERT_In/1 -> V_OUTMON/1, V_OUT/1
  ROLL_In/1 -> R_OUTMON/1, R_OUT/1
  R_OUTMON/1 -> ROLL_Out/1
  V_OUTMON/1 -> VERT_Out/1
  TRANS_In/1 -> T_OUTMON/1, T_OUT/1
  T_OUTMON/1 -> TRANS_Out/1
  LONG_In/1 -> L_OUTMON/1, L_OUT/1
  L_OUTMON/1 -> LONG_Out/1
